simulink model "CiEngineCore"  (R2017b)
settings: Solver=VariableStepAuto  StartTime=0.0  StopTime=inf  RelTol=1e-3  EnableMultiTasking=on
model workspace (MAT data in the model file):
  AFRStoich = 14.6
  AirFilterArea = 0.000962112750162
  AirIntakeVol = 0.0018
  C_eng = 40000
  CompEff = [0.2 0.2 0.2 0.2 0.2 0.2 0.2 0.2 0.2 0.2 0.2 0.2 ... (6000 elements, 60x100)]
  CompMassFlwRate = [0 0.00256701884694 0.00511455880808 0.00766649491749 0.0102195028494 0.0127729401774 0.0153265889731 0.017880362476 0.0204342099213 0.0229881081418 0.0255420430633 0.0280960028754 ... (6000 elements, 60x100)]
  CompPrsRatioBreakPoints = [1 1.02808080808 1.05616161616 1.08424242424 1.11232323232 1.1404040404 1.16848484848 1.19656565657 1.22464646465 1.25272727273 1.28080808081 1.30888888889 1.33696969697 1.36505050505 1.39313131313 1.42121212121 1.44929292929 1.47737373737 1.50545454545 1.53353535354 1.56161616162 1.5896969697 1.61777777778 1.64585858586 1.67393939394 1.70202020202 1.7301010101 1.75818181818 1.78626262626 1.81434343434 1.84242424242 1.87050505051 1.89858585859 1.92666666667 1.95474747475 1.98282828283 2.01090909091 2.03898989899 2.06707070707 2.09515151515 2.12323232323 2.15131313131 2.17939393939 2.20747474747 2.23555555556 2.26363636364 2.29171717172 2.3197979798 2.34787878788 2.37595959596 2.40404040404 2.43212121212 2.4602020202 2.48828282828 2.51636363636 2.54444444444 2.57252525253 2.60060606061 2.62868686869 2.65676767677 2.68484848485 2.71292929293 2.74101010101 2.76909090909 2.79717171717 2.82525252525 2.85333333333 2.88141414141 2.90949494949 2.93757575758 2.96565656566 2.99373737374 3.02181818182 3.0498989899 3.07797979798 3.10606060606 3.13414141414 3.16222222222 3.1903030303 3.21838383838 3.24646464646 3.27454545455 3.30262626263 3.33070707071 3.35878787879 3.38686868687 3.41494949495 3.44303030303 3.47111111111 3.49919191919 3.52727272727 3.55535353535 3.58343434343 3.61151515152 3.6395959596 3.66767676768 3.69575757576 3.72383838384 3.75191919192 3.78]
  CompRefPrs = 101325
  CompRefTemp = 300
  CompSpdBreakPoints = [0 422.344846438 844.689692876 1267.03447648 1689.3794067 2111.72412747 2534.06895296 2956.4139879 3378.75881339 3801.10374361 4223.44825494 4645.79349931 5068.13790593 5490.48294086 5912.8279758 6335.17238241 6757.51762678 7179.86182396 7602.20748721 8024.55231271 8446.89650988 8869.24133538 9291.58699863 9713.9311958 10136.2759166 10558.6216845 10980.9658817 11403.3100789 11825.6558469 12248.0005676 12670.3447648 13092.6904281 13515.0352536 13937.3794507 14359.7246951 14782.0688923 15204.4151839 15626.759381 16049.1046254 16471.4488226 16893.7930198 17316.1382641 17738.4824613 18160.8287529 18583.1729501 19005.5181944 19427.8623916 19850.207636 20272.5518332 20694.8981247 21117.2423219 21539.5865191 21961.9317635 22384.2770078 22806.621205 23228.9654022 23651.3116937 24073.6558909 24496.0011353 24918.3453325]
  CoolantTemp = 310
  Cps = 2
  EgrArea = 0.000314159265359
  EgrCoolantTemp = 360
  EgrEffectiveness = 0.8
  ExhSysArea = 0.000804247719319
  ExhSysVol = 0.0008
  IcEffectiveness = 0.9
  InjSlp = 6.45161290323
  LHV = 47300000
  NCyl = 4
  Pstd = 101325
  Rair = 287.05
  Rexh = 297
  T_cool_start = 355
  T_coolnt_init = 355
  T_coolnt_max = 375
  Tstd = 293.15
  TurbEff = [0.008 0.008 0.008 0.008 0.008 0.008 0.008 0.008 0.008 0.008 0.008 0.008 ... (28800 elements, 60x80x6)]
  TurbMassFlwRate = [7.02000192308e-05 7.02000192308e-05 7.02000192308e-05 7.02000192308e-05 7.02000192308e-05 7.02000192308e-05 7.02000192308e-05 7.02000192308e-05 7.02000192308e-05 7.02000192308e-05 7.02000192308e-05 7.02000192308e-05 ... (28800 elements, 60x80x6)]
  TurbPrsRatioBreakPoints = [1 1.03481012658 1.06962025316 1.10443037975 1.13924050633 1.17405063291 1.20886075949 1.24367088608 1.27848101266 1.31329113924 1.34810126582 1.38291139241 1.41772151899 1.45253164557 1.48734177215 1.52215189873 1.55696202532 1.5917721519 1.62658227848 1.66139240506 1.69620253165 1.73101265823 1.76582278481 1.80063291139 1.83544303797 1.87025316456 1.90506329114 1.93987341772 1.9746835443 2.00949367089 2.04430379747 2.07911392405 2.11392405063 2.14873417722 2.1835443038 2.21835443038 2.25316455696 2.28797468354 2.32278481013 2.35759493671 2.39240506329 2.42721518987 2.46202531646 2.49683544304 2.53164556962 2.5664556962 2.60126582278 2.63607594937 2.67088607595 2.70569620253 2.74050632911 2.7753164557 2.81012658228 2.84493670886 2.87974683544 2.91455696203 2.94936708861 2.98417721519 3.01898734177 3.05379746835 3.08860759494 3.12341772152 3.1582278481 3.19303797468 3.22784810127 3.26265822785 3.29746835443 3.33227848101 3.36708860759 3.40189873418 3.43670886076 3.47151898734 3.50632911392 3.54113924051 3.57594936709 3.61075949367 3.64556962025 3.68037974684 3.71518987342 3.75]
  TurbRackBreakPoints = [0 0.2 0.3 0.5 0.7 1]
  TurbRefPrs = 101325
  TurbRefTemp = 300
  TurbSpdBreakPoints = [0 267.361773363 534.723546727 802.08532009 1069.44709345 1336.80886682 1604.17064018 1871.53241354 2138.89418691 2406.25596027 2673.61773363 2940.979507 3208.34128036 3475.70305372 3743.06482709 4010.42660045 4277.78837381 4545.15014718 4812.51192054 5079.8736939 5347.23546727 5614.59724063 5881.95901399 6149.32078736 6416.68256072 6684.04433408 6951.40610745 7218.76788081 7486.12965417 7753.49142754 8020.8532009 8288.21497426 8555.57674763 8822.93852099 9090.30029435 9357.66206772 9625.02384108 9892.38561444 10159.7473878 10427.1091612 10694.4709345 10961.8327079 11229.1944813 11496.5562546 11763.918028 12031.2798014 12298.6415747 12566.0033481 12833.3651214 13100.7268948 13368.0886682 13635.4504415 13902.8122149 14170.1739883 14437.5357616 14704.897535 14972.2593083 15239.6210817 15506.9828551 15774.3446284]
  TurboInertia = 6e-06
  Vd = 0.0015
  Vexh = 0.000696349540849
  Vint = 0.00286
  cp_air = 1005
  cp_exh = 1005
  f_co = [1.40212981041e-06 1.40212981041e-06 1.6332261526e-06 1.85316257772e-06 2.13933731744e-06 2.5578774362e-06 3.5801963158e-06 5.71066968323e-06 9.06691784867e-06 1.17856264254e-05 1.13266430068e-05 1.17075290539e-05 ... (240 elements, 16x15)]
  f_co2 = [0.0565058276487 0.0565058276487 0.0680775298139 0.0795416117649 0.0927502758383 0.108898516704 0.135970777083 0.163224038089 0.18390566243 0.187824483941 0.180854201863 0.181624048607 ... (240 elements, 16x15)]
  f_exhfrac_n_bpt = [750 1053.57142857 1357.14285714 1660.71428571 1964.28571429 2267.85714286 2571.42857143 2875 3178.57142857 3482.14285714 3785.71428571 4089.28571429 4392.85714286 4696.42857143 5000]
  f_exhfrac_trq_bpt = [0 15 26.4285714286 37.8571428571 49.2857142857 60.7142857143 72.1428571429 83.5714285714 95 106.428571429 117.857142857 129.285714286 140.714285714 152.142857143 163.571428571 175]
  f_fric_temp_bpt = [274 276 278 280 282 284 286 288 290 292 294 296 298 300 302 304 306 308 310 312 314 316 318 320 322 324 326 328 330 332 334 336 338 340 342 344 346 348 350 352 354 356 358 360 362 364 366 368 370 372 374 376 378 380]
  f_fric_temp_mod = [3.96 3.22 2.56 2.26 2.11 2 1.9 1.83 1.76 1.7 1.65 1.6 1.55 1.49 1.44 1.41 1.38 1.35 1.32 1.3 1.27 1.25 1.24 1.21 1.2 1.18 1.16 1.15 1.13 1.12 1.11 1.1 1.09 1.08 1.07 1.06 1.05 1.05 1.04 1.03 1.02 1.02 1.01 1.01 1 1 1 0.999 0.997 0.995 0.993 0.991 0.989 0.987]
  f_hc = [1.08896576916e-07 1.08896576916e-07 1.53414498342e-07 2.00715453959e-07 2.48790869997e-07 2.97869368014e-07 3.52504999231e-07 4.04349945817e-07 4.52780325277e-07 4.91342452993e-07 4.91996758973e-07 4.96487624267e-07 ... (240 elements, 16x15)]
  f_nox = [9.38886565825e-05 9.38886565825e-05 0.000158278744526 0.000381657424268 0.00062836202089 0.000865097048745 0.000965103000667 0.00083216127124 0.00082959112316 0.00143554359074 0.00196340813932 0.0020351396325 ... (240 elements, 16x15)]
  f_nv = [0.954646224834 0.927678310575 0.901063682417 0.875710037198 0.852450535311 0.831986822876 0.814844392337 0.80134438932 0.791593989181 0.785495277781 0.782770492696 0.782999798686 ... (450 elements, 30x15)]
  f_nv_n_bpt = [1000 1285.71428571 1571.42857143 1857.14285714 2142.85714286 2428.57142857 2714.28571429 3000 3285.71428571 3571.42857143 3857.14285714 4142.85714286 4428.57142857 4714.28571429 5000]
  f_nv_prs_bpt = [95 100.344827586 105.689655172 111.034482759 116.379310345 121.724137931 127.068965517 132.413793103 137.75862069 143.103448276 148.448275862 153.793103448 159.137931034 164.482758621 169.827586207 175.172413793 180.517241379 185.862068966 191.206896552 196.551724138 201.896551724 207.24137931 212.586206897 217.931034483 223.275862069 228.620689655 233.965517241 239.310344828 244.655172414 250]
  f_t_exh = [358.711368346 429.963145924 497.987869771 559.016510887 625.497016294 690.207854611 731.780908025 749.899407528 764.155922317 789.797182974 824.513264157 858.92580636 ... (240 elements, 16x15)]
  f_t_exh_f_bpt = [0 3.57 6.855 10.14 13.425 16.71 19.995 23.28 26.565 29.85 33.135 36.42 39.705 42.99 46.275 49.56]
  f_t_exh_n_bpt = [1000 1285.71428571 1571.42857143 1857.14285714 2142.85714286 2428.57142857 2714.28571429 3000 3285.71428571 3571.42857143 3857.14285714 4142.85714286 4428.57142857 4714.28571429 5000]
  f_tq_apc_bpt = [94.6146459029 109.976602506 125.338559109 140.700515712 156.062472315 171.424428919 186.786385522 202.148342125 217.510298728 232.872255331 248.234211934 263.596168537 278.958125141 294.320081744 309.682038347]
  f_tq_apc_mod = [0.999715885044 0.999538569407 0.999259905514 0.998809242093 0.998358578671 0.997880679846 0.997234389999 0.996588100153 0.995941810306 0.99547925674 0.995035391789 0.994591526839 ... (240 elements, 15x16)]
  f_tq_fric = [0  8.35  9.18  10  10.9  11.8  12.8  13.7  14.7  15.8  16.8  17.8  18.9  20  21.1  22.2; 0  8.35  9.18  10  10.9  11.8  12.8  13.7  14.7  15.8  16.8  17.8  18.9  20  21.1  22.2; 0  8.57  9.36  10.2  11.1  12  12.9  13.9  14.9  16  17  18.1  19.2  20.2  21.3  22.4; 0  8.79  9.56  10.4  11.2  12.2  13.1  14.1  15.2  16.2  17.3  18.4  19.5  20.6  21.6  22.7; 0  8.99  9.74  10.6  11.5  12.4  13.4  14.4  15.4  16.5  17.6  18.7  19.8  20.9  22  23.1; 0  9.19  9.94  10.8  11.7  12.7  13.7  14.7  15.8  16.8  17.9  19  20  21.1  22.3  23.4; 0  9.42  10.2  11  12  13.1  14.1  15.2  16.2  17.3  18.3  19.3  20.4  21.5  22.6  23.7; 0  9.7  10.4  11.3  12.4  13.5  14.6  15.7  16.8  17.9  18.9  19.9  21  22  23.1  24.1; 0  9.78  10.6  11.6  12.6  13.8  15  16.1  17.3  18.4  19.5  20.5  21.6  22.6  23.7  24.7; 0  9.84  10.8  11.7  12.8  13.9  15.1  16.3  17.5  18.6  19.7  20.8  21.9  23  24  25.1; 0  9.92  10.9  11.9  12.9  14.1  15.3  16.4  17.6  18.6  19.7  20.8  21.9  23  24.1  25.2; 0  10  11  12  13.1  14.3  15.5  16.7  17.8  18.8  19.9  20.9  22  23.1  24.2  25.4; 0  10.1  11.2  12.2  13.3  14.5  15.7  16.9  18.1  19.1  20.2  21.2  22.2  23.3  24.4  25.6; 0  10.3  11.3  12.3  13.4  14.6  15.7  16.9  18.1  19.2  20.3  21.3  22.4  23.4  24.6  25.7; 0  10.4  11.4  12.5  13.6  14.7  15.8  17  18.1  19.2  20.3  21.4  22.5  23.6  24.7  25.9; 0  10.5  11.6  12.6  13.7  14.8  15.9  17  18.2  19.3  20.4  21.5  22.6  23.7  24.8  26]
  f_tq_inr = [0 18.932941535 39.3255223176 57.8807366655 73.6414164249 90.1575991353 102.879416349 112.92944314 130.905512841 149.615511709 168.234721026 187.879026911 ... (256 elements, 16x16)]
  f_tq_inr_f_bpt = [0 3.57 6.855 10.14 13.425 16.71 19.995 23.28 26.565 29.85 33.135 36.42 39.705 42.99 46.275 49.56]
  f_tq_inr_n_bpt = [0 1000 1285.71428571 1571.42857143 1857.14285714 2142.85714286 2428.57142857 2714.28571429 3000 3285.71428571 3571.42857143 3857.14285714 4142.85714286 4428.57142857 4714.28571429 5000]
  f_tq_mainsoi_bpt = [-15 -13.7142857143 -12.4285714286 -11.1428571429 -9.85714285714 -8.57142857143 -7.28571428571 -6 -4.71428571429 -3.42857142857 -2.14285714286 -0.857142857143 0.428571428571 1.71428571429 3]
  f_tq_mainsoi_mod = [0.81078150005 0.827839263513 0.848673573925 0.874587588348 0.900164013454 0.923298328972 0.948048831471 0.970618714872 0.98831830141 0.997452724955 1 1 ... (240 elements, 15x16)]
  f_tq_map_bpt = [94.6146459029 109.976602506 125.338559109 140.700515712 156.062472315 171.424428919 186.786385522 202.148342125 217.510298728 232.872255331 248.234211934 263.596168537 278.958125141 294.320081744 309.682038347]
  f_tq_map_mod = [0.882177094009 0.934851504719 0.96634483908 0.97127123182 0.962954413121 0.952665164101 0.94513861625 0.942129377179 0.94335561462 0.947447812134 0.952949052459 0.958725491494 ... (240 elements, 15x16)]
  f_tq_mat_bpt = [35 42.8571428571 50.7142857143 58.5714285714 66.4285714286 74.2857142857 82.1428571429 90 97.8571428571 105.714285714 113.571428571 121.428571429 129.285714286 137.142857143 145]
  f_tq_mat_mod = [0.979193935333 0.989700620258 0.997707737278 1 0.992841543128 0.973230182048 0.94195882355 0.902873432246 0.86074346216 0.81947608235 0.779242235611 0.739783745312 ... (240 elements, 15x16)]
  f_tq_nf = [nan nan nan nan nan nan nan nan nan nan nan nan ... (256 elements, 16x16)]
  f_tq_nf_f_bpt = [0 3.57 6.855 10.14 13.425 16.71 19.995 23.28 26.565 29.85 33.135 36.42 39.705 42.99 46.275 49.56]
  f_tq_nf_n_bpt = [0 1000 1285.71428571 1571.42857143 1857.14285714 2142.85714286 2428.57142857 2714.28571429 3000 3285.71428571 3571.42857143 3857.14285714 4142.85714286 4428.57142857 4714.28571429 5000]
  f_tq_pump = [0  1  1  1.14  1.4  1.7  1.98  2.25  2.57  2.99  3.52  4.17  4.97  5.8  6.65  7.52; 0  1  1  1.14  1.4  1.7  1.98  2.25  2.57  2.99  3.52  4.17  4.97  5.8  6.65  7.52; 0  1  1  1.14  1.39  1.7  1.95  2.18  2.44  2.79  3.23  3.8  4.58  5.38  6.2  6.83; 0  1  1  1.11  1.32  1.7  2.05  2.37  2.7  3.03  3.4  3.83  4.45  5.19  6.02  6.74; 0  1  1  1.05  1.18  1.57  1.99  2.46  2.99  3.54  4.05  4.5  4.93  5.45  6.04  6.69; 0  1  1  1  1.03  1.31  1.64  2.04  2.6  3.3  4.01  4.67  5.2  5.73  6.3  7.01; 0  1  1  1.06  1.23  1.83  2.31  2.73  3.11  3.53  3.95  4.35  4.75  5.27  5.94  6.98; 0  1  1  1.21  1.7  3.02  4.17  5.18  5.95  6.49  6.85  6.98  6.84  6.8  6.92  7.67; 0  1  1  1  1.18  2.66  4.22  5.82  7.42  8.93  10.2  11.1  11.3  11.2  10.9  10.9; 0  1  1  1  1.06  1.51  2.69  4.26  6.02  7.9  9.71  11.4  12.4  13.2  13.6  13.9; 0  1  1  1  1  1  1.81  3.05  4.51  5.87  7.14  8.31  9.49  10.7  12.1  13.4; 0  1  1  1  1  1  1.43  2.28  3.79  4.97  5.92  6.63  7.49  8.67  10.2  12.2; 0  1  1  1  1  1  1.13  1.68  3.34  4.75  5.91  6.75  7.6  8.75  10.3  12.4; 0  1  1  1  1  1  1  1.38  2.91  4.49  5.87  6.9  7.77  9.05  10.8  13; 0  1  1  1  1  1  1  1.35  2.73  4.29  5.79  7.11  8.33  9.8  11.5  13.8; 0  1  1  1  1  1  1  1.36  2.78  4.33  5.88  7.38  8.91  10.6  12.4  14.6]
  tau_cool = 3000
undefined symbols (not defined in the file): ThrAngToC
libraries: autolibfundflw x11, autolibboost x3, autolibcoreeng x1, simulink x1
(part 1 of 2)
settings Model: ModifiedByFormat=The MathWorks, Inc.  Creator=The MathWorks, Inc.  LastModifiedBy=The MathWorks, Inc.
settings DataIOCC: DSMLogging=off
settings CodeAppCC: StateflowObjectComments=on
settings GRTTargetCC: TargetLangStandard=C89/C90 (ANSI)
settings ConfigComp: CovMetricSettings=dsw  CovHtmlReporting=on  CovSaveCumulativeToWorkspaceVar=on  CovSaveSingleToWorkspaceVar=on  CovShowResultsExplorer=off  CovExternalEMLEnable=off
settings SimscapeCC: SimscapeNormalizeSystem=off  SimscapeNominalValues={1, 'bar'; 1, 'cm^3/s'; 1, 'bar*kg/s'; 1, 'kJ/kg'; 1, 'kW'; }

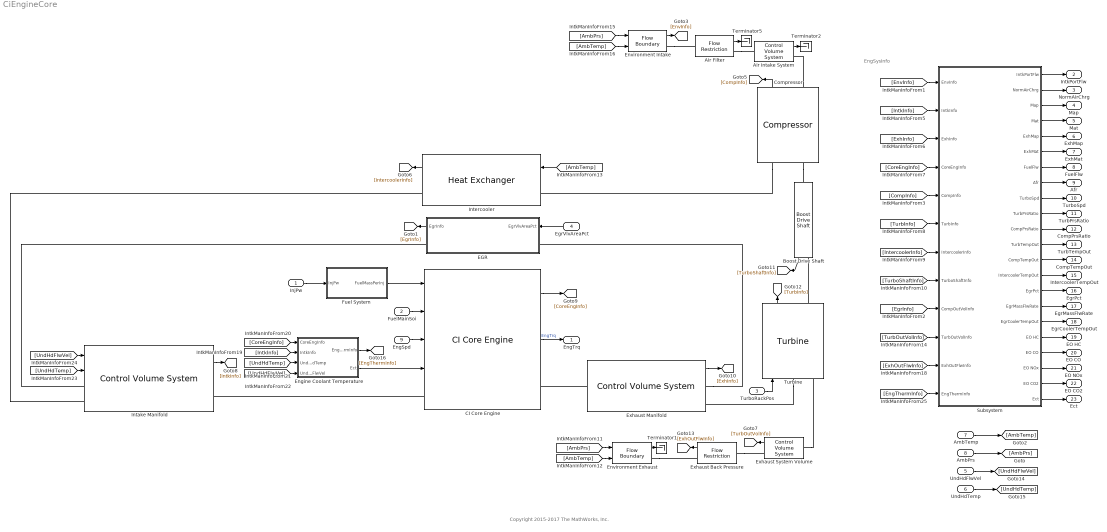
== system CiEngineCore ==
  note: EngSysInfo
  note: Copyright 2015-2017 The MathWorks, Inc.
  InjPw : Inport
  FuelMainSoi : Inport  Port=2
  TurboRackPos : Inport  Port=3
  EgrVlvAreaPct : Inport  Port=4
  UndHdFlwVel : Inport  Port=5
  UndHdTemp : Inport  Port=6
  AmbTemp : Inport  Port=7
  AmbPrs : Inport  Port=8
  EngSpd : Inport  Port=9
  Air Filter : autolibfundflw/Flow Restriction  AreaPopup=Constant  ImageTypePopup=Cold  gamma=cp_air/(cp_air-Rair)  R=Rair  Plim=0.9  Aorf_cnst=AirFilterArea  Cd_cnst=1  Cd_ext=1  Dthr=50  ThrCd=[0.001; 0.735]  ThrAngBpts=[0; 90]
      settings: SourceProductName=Powertrain Blockset  SourceProductBaseCode=PW
  Air Intake System : autolibfundflw/Control Volume System  NumInletPorts=1  NumOutletPorts=1  HeatTransferModelPopup=Constant  ImageTypePopup=Cold  Vch=AirIntakeVol  Pinit=101325  Tinit=298  R=Rair  cp=cp_air  q_he=0  ext_tbl=[40 160 740 2000]  ext_bpts=linspace(0,180,4)  Aext_conv=0.125  m_wall=7  cp_wall=900  Tmass=293.15  Dext_cond=0.004  Aext_cond=0.003  kext=25  Dint_cond=0.004  Aint_cond=0.003  kint=25  int_tbl=[40 160 740 2000]  int_bpts=linspace(0.0020,0.1100,4)  Aint_conv=0.125
      settings: SourceProductName=Powertrain Blockset  SourceProductBaseCode=PW
  Boost Drive Shaft : autolibboost/Boost Drive Shaft  ShaftConfigPopup=Turbocharger  AddTrqTypePopup=No external torque  J_shaft=TurboInertia  w_0=5000*pi/30  w_min=1  w_max=1e6  eta_mech=1
      settings: SourceProductName=Powertrain Blockset  SourceProductBaseCode=PW
  CI Core Engine : autolibcoreeng/CI Core Engine  TrqOptionPopup=Torque Structure  NCyl=NCyl  Cps=Cps  Vd=Vd  Rair=Rair  Pstd=Pstd  Tstd=Tstd  f_nv=f_nv  f_nv_prs_bpt=f_nv_prs_bpt  f_nv_n_bpt=f_nv_n_bpt  f_tq_nf=f_tq_nf  f_tq_nf_f_bpt=f_tq_nf_f_bpt  f_tq_nf_n_bpt=f_tq_nf_n_bpt  f_tq_inr=f_tq_inr  f_tq_fric=f_tq_fric  f_fric_temp_mod=f_fric_temp_mod  f_fric_temp_bpt=f_fric_temp_bpt  f_tq_pump=f_tq_pump  f_tq_inr_f_bpt=f_tq_inr_f_bpt  f_tq_inr_n_bpt=f_tq_inr_n_bpt  f_tq_mainsoi_mod=f_tq_mainsoi_mod  f_tq_mainsoi_bpt=f_tq_mainsoi_bpt  f_tq_mat_mod=f_tq_mat_mod  f_tq_mat_bpt=f_tq_mat_bpt  f_tq_map_mod=f_tq_map_mod  f_tq_map_bpt=f_tq_map_bpt  f_tq_apc_mod=f_tq_apc_mod  f_tq_apc_bpt=f_tq_apc_bpt  f_t_exh=f_t_exh  f_t_exh_f_bpt=f_t_exh_f_bpt  f_t_exh_n_bpt=f_t_exh_n_bpt  cp_exh=cp_exh  CO2EmissionsCheckbox=on  COEmissionsCheckbox=on  NOxEmissionsCheckbox=on  HCEmissionsCheckbox=on  PMEmissionsCheckbox=off  f_CO2_frac=f_co2  f_CO_frac=f_co  f_HC_frac=f_hc  f_NOx_frac=f_nox  f_PM_frac=zeros(size(f_nox))  f_exhfrac_n_bpt=f_exhfrac_n_bpt  f_exhfrac_trq_bpt=f_exhfrac_trq_bpt  afr_stoich=AFRStoich
      settings: SourceProductName=Powertrain Blockset  SourceProductBaseCode=PW
  Compressor : autolibboost/Compressor  mdot_corr_tbl=CompMassFlwRate  eta_comp_tbl=CompEff  w_corr_bpts1=CompSpdBreakPoints  Pr_bpts2=CompPrsRatioBreakPoints  T_ref=CompRefTemp  P_ref=CompRefPrs  R=Rair  cp=cp_air
      settings: SourceProductName=Powertrain Blockset  SourceProductBaseCode=PW
  EGR : Subsystem
  Engine Coolant Temperature : Subsystem
  Environment Exhaust : autolibfundflw/Flow Boundary  PrsTempSrcPopup=External input  ImageTypePopup=Hot  Pcnst=101325  Tcnst=298.15  cp=cp_air
      settings: SourceProductName=Powertrain Blockset  SourceProductBaseCode=PW
  Environment Intake : autolibfundflw/Flow Boundary  PrsTempSrcPopup=External input  ImageTypePopup=Cold  Pcnst=101325  Tcnst=298.15  cp=cp_air
      settings: SourceProductName=Powertrain Blockset  SourceProductBaseCode=PW
  Exhaust Back Pressure : autolibfundflw/Flow Restriction  AreaPopup=Constant  ImageTypePopup=Hot  gamma=cp_exh/(cp_exh-Rexh)  R=Rexh  Plim=0.9  Aorf_cnst=ExhSysArea  Cd_cnst=1  Cd_ext=1  Dthr=50  ThrCd=[0.001; 0.735]  ThrAngBpts=[0; 90]
      settings: SourceProductName=Powertrain Blockset  SourceProductBaseCode=PW
  Exhaust Manifold : autolibfundflw/Control Volume System  NumInletPorts=1  NumOutletPorts=2  HeatTransferModelPopup=Constant  ImageTypePopup=Hot  Vch=Vexh  Pinit=101325  Tinit=298  R=Rexh  cp=cp_exh  q_he=0  ext_tbl=[40 160 740 2000]  ext_bpts=linspace(0,180,4)  Aext_conv=0.125  m_wall=7  cp_wall=900  Tmass=293.15  Dext_cond=0.004  Aext_cond=0.003  kext=25  Dint_cond=0.004  Aint_cond=0.003  kint=25  int_tbl=[40 160 740 2000]  int_bpts=linspace(0.0020,0.1100,4)  Aint_conv=0.125
      settings: SourceProductName=Powertrain Blockset  SourceProductBaseCode=PW
  Exhaust System Volume : autolibfundflw/Control Volume System  NumInletPorts=1  NumOutletPorts=1  HeatTransferModelPopup=Constant  ImageTypePopup=Hot  Vch=ExhSysVol  Pinit=101325  Tinit=298  R=Rexh  cp=cp_exh  q_he=0  ext_tbl=[40 160 740 2000]  ext_bpts=linspace(0,180,4)  Aext_conv=0.125  m_wall=7  cp_wall=900  Tmass=293.15  Dext_cond=0.004  Aext_cond=0.003  kext=25  Dint_cond=0.004  Aint_cond=0.003  kint=25  int_tbl=[40 160 740 2000]  int_bpts=linspace(0.0020,0.1100,4)  Aint_conv=0.125
      settings: SourceProductName=Powertrain Blockset  SourceProductBaseCode=PW
  Fuel System : Subsystem
  Intake Manifold : autolibfundflw/Control Volume System  NumInletPorts=2  NumOutletPorts=1  HeatTransferModelPopup=External wall convection  ImageTypePopup=Cold  Vch=Vint  Pinit=101325  Tinit=298  R=Rair  cp=cp_air  q_he=0  ext_tbl=[40 160 740 2000]  ext_bpts=linspace(0,180,4)  Aext_conv=0.125  m_wall=7  cp_wall=900  Tmass=293.15  Dext_cond=0.004  Aext_cond=0.003  kext=25  Dint_cond=0.004  Aint_cond=0.003  kint=25  int_tbl=[40 160 740 2000]  int_bpts=linspace(0.0020,0.1100,4)  Aint_conv=0.125
      settings: SourceProductName=Powertrain Blockset  SourceProductBaseCode=PW
  Intercooler : autolibfundflw/Heat Exchanger  EffctModelPopup=Constant  CoolTempInputPopup=External input  ImageTypePopup=Intercooler  ep_cnst=IcEffectiveness  T_cool_cnst=CoolantTemp  cp=cp_air
      settings: SourceProductName=Powertrain Blockset  SourceProductBaseCode=PW
  Subsystem : Subsystem
  Terminator1 : Terminator
  Terminator2 : Terminator
  Terminator5 : Terminator
  Turbine : autolibboost/Turbine  TurbTypePopup=Variable geometry  WgIncludeCheckbox=off  mdot_corrfx_tbl=TurbMassFlwRate  mdot_corrvr_tbl=TurbMassFlwRate  eta_turbfx_tbl=TurbEff  eta_turbvr_tbl=TurbEff  w_corrfx_bpts1=TurbSpdBreakPoints  w_corrvr_bpts2=TurbSpdBreakPoints  Pr_fx_bpts2=TurbPrsRatioBreakPoints  Pr_vr_bpts2=TurbPrsRatioBreakPoints  L_rack_bpts3=TurbRackBreakPoints  T_ref=TurbRefTemp  P_ref=TurbRefPrs  mdot_thresh=1e-6  A_wgopen=WgArea  Plim_wg=.99  R=Rexh  cp=cp_exh
      settings: SourceProductName=Powertrain Blockset  SourceProductBaseCode=PW
  EngTrq : Outport
  IntkPortFlw : Outport  Port=2
  NormAirChrg : Outport  Port=3
  Map : Outport  Port=4
  Mat : Outport  Port=5
  ExhMap : Outport  Port=6
  ExhMat : Outport  Port=7
  FuelFlw : Outport  Port=8
  Afr : Outport  Port=9
  TurboSpd : Outport  Port=10
  TurbPrsRatio : Outport  Port=11
  CompPrsRatio : Outport  Port=12
  TurbTempOut : Outport  Port=13
  CompTempOut : Outport  Port=14
  IntercoolerTempOut : Outport  Port=15
  EgrPct : Outport  Port=16
  EgrMassFlwRate : Outport  Port=17
  EgrCoolerTempOut : Outport  Port=18
  EO HC : Outport  Port=19
  EO CO : Outport  Port=20
  EO NOx : Outport  Port=21
  EO CO2 : Outport  Port=22
  Ect : Outport  Port=23
  wires:
  EgrVlvAreaPct/1 -> EGR/1(EgrVlvAreaPct)
  EGR/1(EgrInfo) -> [EgrInfo]
  EngSpd/1 -> CI Core Engine/3
  [AmbTemp] -> Intercooler/1
  [AmbTemp] -> Environment Exhaust/2
  [AmbPrs] -> Environment Exhaust/1
  Environment Intake/1 -> [EnvInfo]
  AmbPrs/1 -> [AmbPrs]
  AmbTemp/1 -> [AmbTemp]
  Turbine/1 -> [TurbInfo]
  Boost Drive Shaft/1 -> [TurboShaftInfo]
  Exhaust Manifold/1 -> [ExhInfo]
  CI Core Engine/1 -> [CoreEngInfo]
  Intake Manifold/1 -> [IntkInfo]
  Compressor/1 -> [CompInfo]
  CI Core Engine/2 -> EngTrq/1  "EngTrq"
  Intercooler/1 -> [IntercoolerInfo]
  Air Filter/1 -> Terminator5/1
  Air Intake System/1 -> Terminator2/1
  Exhaust System Volume/1 -> [TurbOutVolInfo]
  Exhaust Back Pressure/1 -> [ExhOutFlwInfo]
  Environment Exhaust/1 -> Terminator1/1
  [AmbPrs] -> Environment Intake/1
  [AmbTemp] -> Environment Intake/2
  [EnvInfo] -> Subsystem/1(EnvInfo)
  [IntkInfo] -> Subsystem/2(IntkInfo)
  [ExhInfo] -> Subsystem/3(ExhInfo)
  [CoreEngInfo] -> Subsystem/4(CoreEngInfo)
  [CompInfo] -> Subsystem/5(CompInfo)
  [TurbInfo] -> Subsystem/6(TurbInfo)
  [IntercoolerInfo] -> Subsystem/7(IntercoolerInfo)
  [TurboShaftInfo] -> Subsystem/8(TurboShaftInfo)
  Subsystem/1(IntkPortFlw) -> IntkPortFlw/1
  Subsystem/5(ExhMap) -> ExhMap/1
  Subsystem/4(Mat) -> Mat/1
  Subsystem/3(Map) -> Map/1
  Subsystem/6(ExhMat) -> ExhMat/1
  Subsystem/7(FuelFlw) -> FuelFlw/1
  Subsystem/8(Afr) -> Afr/1
  Subsystem/2(NormAirChrg) -> NormAirChrg/1
  Subsystem/9(TurboSpd) -> TurboSpd/1
  Subsystem/10(TurbPrsRatio) -> TurbPrsRatio/1
  Subsystem/11(CompPrsRatio) -> CompPrsRatio/1
  Subsystem/12(TurbTempOut) -> TurbTempOut/1
  Subsystem/13(CompTempOut) -> CompTempOut/1
  Subsystem/14(IntercoolerTempOut) -> IntercoolerTempOut/1
  [TurbOutVolInfo] -> Subsystem/10(TurbOutVolInfo)
  [EgrInfo] -> Subsystem/9(CompOutVolInfo)
  Subsystem/15(EgrPct) -> EgrPct/1
  Subsystem/16(EgrMassFlwRate) -> EgrMassFlwRate/1
  Subsystem/17(EgrCoolerTempOut) -> EgrCoolerTempOut/1
  FuelMainSoi/1 -> CI Core Engine/2
  [ExhOutFlwInfo] -> Subsystem/11(ExhOutFlwInfo)
  Subsystem/18(EO HC) -> EO HC/1
  Subsystem/19(EO CO) -> EO CO/1
  Subsystem/20(EO NOx) -> EO NOx/1
  Subsystem/21(EO CO2) -> EO CO2/1
  InjPw/1 -> Fuel System/1(InjPw)
  Fuel System/1(FuelMassPerInj) -> CI Core Engine/1
  TurboRackPos/1 -> Turbine/1
  Subsystem/22(Ect) -> Ect/1
  [UndHdTemp] -> Engine Coolant Temperature/3(UndHdTemp)
  [IntkInfo] -> Engine Coolant Temperature/2(IntkInfo)
  [UndHdFlwVel] -> Engine Coolant Temperature/4(UndHdFlwVel)
  [CoreEngInfo] -> Engine Coolant Temperature/1(CoreEngInfo)
  UndHdFlwVel/1 -> [UndHdFlwVel]
  UndHdTemp/1 -> [UndHdTemp]
  [UndHdTemp] -> Intake Manifold/2
  [UndHdFlwVel] -> Intake Manifold/1
  Engine Coolant Temperature/1(EngThermInfo) -> [EngThermInfo]
  Engine Coolant Temperature/2(Ect) -> CI Core Engine/4
  [EngThermInfo] -> Subsystem/12(EngThermInfo)
  connections:
  Exhaust Manifold/LConn1 -- CI Core Engine/RConn1
  Intake Manifold/LConn1 -- EGR/RConn1
  Exhaust Manifold/RConn1 -- EGR/LConn1
  Compressor/LConn1 -- Intercooler/LConn1
  Compressor/LConn2 -- Boost Drive Shaft/LConn1
  Turbine/RConn1 -- Boost Drive Shaft/RConn1
  Exhaust Back Pressure/LConn1 -- Exhaust System Volume/RConn1
  CI Core Engine/LConn1 -- Intake Manifold/RConn1
  Environment Intake/RConn1 -- Air Filter/LConn1
  Environment Exhaust/RConn1 -- Exhaust Back Pressure/RConn1
  Compressor/RConn1 -- Air Intake System/RConn1
  Intercooler/RConn1 -- Intake Manifold/LConn2
  Turbine/LConn1 -- Exhaust Manifold/RConn2
  Exhaust System Volume/LConn1 -- Turbine/LConn2
  Air Filter/RConn1 -- Air Intake System/LConn1
